simulink model "P2_SIL_Model_Diag"  (R2016a)
settings: Solver=ode2  StartTime=0.0  StopTime=Cycle_End  RelTol=1e-3
undefined symbols (not defined in the file): air, APP1_OOR, APP2_OOR, APP_Conversion_IN, APP_Mismatch, bms_inletair_temp, bms_maxchargecurrent, bms_maxdischargecurrent, BMS_Notfallkuehlung, BPP_Flt, cal, clt, ClutchEngag, CrankRequest, dcdc, eng, Engine, EngOverTemp, ENGTRQ_MSMCH_Degraded_CP, ENGTRQ_MSMCH_ErrCritical_CP, ENGTRQ_MSMCH_LimpHome_CP, EngTrqMismatch, env, ess, ESS, ESSOverTemp, fd, FFD, g, gb, Grade, IMG, KeyPos_Flt, KeyPosition, lib_APP_Conversion_IN, lib_ESS_plant_V1_2, lib_OBC_Manager, LossCAN, max_vehicle_rad_air_flow, MCUOverTemp, mot, MotDirMismatch, MotOverTemp, MotTrqMismatch, mph2kph, mph2ms, NeutralGear, obc, OBC_Manager, ParkGear, PRNDL_Flt, ReverseGear, RFD, rho, ShiftLeverPosition, sigbuilder_block, Speed, t_amb, time, tloop ... (+2)
libraries: simulink x104, EC2_libraries x12, Diagnostic x11, lib_CANerror_Detect x3, Utility x1
(part 11 of 11)

== stateflow chart P2_SIL_Model_Diag/Controller/HSC/Powertrain Manager/PowertrainSUSD/Motor Wake up // Shutdown ==
  state MCU_Restart [commented out]
    en:MCU_State = 10;
    MCU_Wake = 0;
    Fault_Counter++;
    during: timer++;
  state MCU_Startup
    state MCU_Wake
      en:MCU_State = 0;
      MCU_Wake = 1;
      MCUFault = 0;
      %Inverter_Enable = 0;
      Inverter_Discharge=0;
      MCU_ShtdwnRdy=0;
      Fault_Counter = 0;
    state MCU_Fault_1
      en:MCU_State = -1;
      MCUFault = 1;
    state MCU_Running
      en:MCU_State =3;
    state MCU_Enable
      en:MCU_State = 2;
      %Inverter_Enable = 1;
      during: timer++;
    state MCU_Ready
      en:MCU_State = 1;
    (default) -> MCU_Wake
    (junction 244) -> MCU_Fault_1 [order 2] : after(10,sec)
    (junction 244) -> MCU_Running [order 1] : [Inverter_Enabled]
    MCU_Enable -> (junction 244)
    MCU_Wake -> MCU_Ready : [CAN_Acc]
    MCU_Ready -> MCU_Enable : [RdyToDrv&&EnableInverter]
        | {timer = 0;}
  state MCU_Shutdown
    state MCU_Disable
      en:MCU_State = 8;
      during: timer++;
    state MCU_RdyForShtDwn
      en:MCU_State = 6;
      MCU_ShtdwnRdy=1;
    state MCU_Discharge_Bus
      en:MCU_State = 7;
      Inverter_Discharge=1;
    state MCU_Shtdwn_Cmplt
      en:MCU_State = 9;
      MCU_Wake = 0;
    state MCU_Fault_3
      en:MCU_State = -3;
      MCUFault = 1;
    (default) -> MCU_RdyForShtDwn : {timer = 0;}
    MCU_RdyForShtDwn -> MCU_Discharge_Bus : [HVDischarge]
    MCU_Discharge_Bus -> MCU_Disable : [!HVDischarge &&!EnableInverter]
        | {timer=0;}
    MCU_Disable -> (junction 247)
    (junction 247) -> MCU_Fault_3 [order 2] : after(10,sec)
    (junction 247) -> MCU_Shtdwn_Cmplt [order 1] : [!Inverter_Enabled]
  MCU_Restart -> MCU_Startup [commented out] : [timer > Restart_Time]
      | {timer = 0;}
  MCU_Startup -> MCU_Restart [commented out] : [(MCU_State==3 && !Inverter_Enabled || MCU_State==-1) && Fault_Counter<6]
      | {timer = 0;}
  MCU_Shutdown -> MCU_Startup : [RdyToDrv || RdyToChg]
  MCU_Startup -> MCU_Shutdown : [!RdyToDrv && !RdyToChg && Motor_Current < MaxShtdwnCrnt]
  (default) -> MCU_Shutdown
  data: MCU_State output int8; MCU_ShtdwnRdy output boolean; MCUFault output boolean; MCU_Wake output boolean; Inverter_Discharge output boolean; Inverter_Enable output boolean; RdyToDrv input boolean; RdyToChg input boolean; HVDischarge input boolean; Inverter_Response_Time input double; Restart_Time input double; MaxShtdwnCrnt input double; Inverter_Enabled input boolean; timer local double; Fault_Counter local double; Motor_Current input; CAN_Acc input boolean; EnableInverter input

== stateflow chart P2_SIL_Model_Diag/Controller/HSC/Powertrain Manager/Torque Distribution/Supervisory  Control  Logic1 ==
  state VehOffOrAcc
    en:
    powerMode = 0;
    EnablePrplsn = 0;
    HV_Req=0;
    closeMaincReq=0;
  state VehOn
    en:
    powerMode = 1;
    HV_Req=1;
    closeMaincReq = 1;
  state VehShutdown
    en:
    powerMode = 1;
    EnablePrplsn = 0;
    EngOnReq = 0;
    MotTrqReq = 0;
    EngAppReq = 0;
    EnableInverter=0;
  state EnablePropulsion
    en:
    EnablePrplsn = 1;
    EnableInverter = 1;
  state VehReady
    en:
    powerMode = 2;
    note: CD Limited
        | Engine Limited
    note: Fault detected?
    state Transition2
      en:
      MotTrqReq = 0;
      EngAppReq = 0;
      ClutchEngage = 1;
      state EngApp = SyncCtrl(EngSpeed,MotorSpeed) [function]
      state EngStart
        en: EngOnReq = 1;
      (default) -> VehReady.Transition2.EngStart : [VehicleSpeed < 1 && TransEstGear == 15]
    state CD_Limited
      en:
      EngOnReq = 0;
      mode=6;
      du:
      MotTrqReq = MotTrqCalc1(drvAPP,BrkPdlPos,VehicleSpeed,ShftLvrPos,MotSpd,DrvIntdAxleTrq,TransRatio,MotTrqMismchDegraded,MotTrqMismchLimp,essTempRange,MCUTempRange,MotorTempRange);
      EngAppReq = 0;
      state T = MotTrqCalc1(APP,BPP,VehSpd,ShftLvrPos,MotSpeed,DrvIntdAxleTrq,TransRatio,MotTrqMismchDegraded,MotTrqMismchLimp,essTempRange,MCUTempRange,MotorTempRange) [function]
    state CD_Mode
      en:
      EngOnReq = 0;
      mode=1;
      du:
      MotTrqReq = MotTrqCalc1(drvAPP,BrkPdlPos,VehicleSpeed,ShftLvrPos,MotSpd,DrvIntdAxleTrq,TransRatio,eSystemStatus);
      EngAppReq = 0;
      state T = MotTrqCalc(APP,BPP,VehSpd,Shifter,MotSpeed) [function] [commented out]
      state T = MotTrqCalc1(APP,BPP,VehSpd,ShftLvrPos,MotSpeed,DrvIntdAxleTrq,TransRatio,eSystemStatus) [function]
    state Sport_Mode
      en:
      mode=4;
      EngOnReq = 1;
      EngTrq = 0;
      du:
      MotTrqReq = MotTrqCalc(drvAPP,BrkPdlPos,VehicleSpeed,ShftLvrPos,MotSpd,DrvIntdAxleTrq,TransRatio);
      EngTrq = EngTrqCalc(drvAPP,EngSpd,ShftLvrPos,DrvIntdAxleTrq,TransRatio);
      EngAppReq = EngTrq2EngApp(EngTrq);
      state T = MotTrqCalc(APP,BPP,VehSpd,Shifter,MotSpeed,DrvIntdAxleTrq,TransRatio) [function]
      state T = EngTrqCalc(APP,EngSpeed,Shifter,DrvIntdAxleTrq,TransRatio) [function]
      state APP = EngTrq2EngApp(Trq) [function]
    state Transition
      en:
      MotTrqReq = 0;
      EngAppReq = 0;
      state EngStart1
        en: EngOnReq = 1;
      state EngApp = SyncCtrl(EngSpeed,MotorSpeed) [function]
      state EngageClutch
        en:
        ClutchEngage = 1;
      state EngSpdSync
        du:
        EngAppReq = SyncCtrl(EngSpd,MotSpd);
      state EngStart
        en: EngOnReq = 1;
      state EngageClutch1
        en:
        ClutchEngage = 1;
      (default) -> (junction 148)
      (junction 148) -> VehReady.Transition.EngStart1 [order 2] : [VehicleSpeed >= 1]
      (junction 148) -> VehReady.Transition.EngageClutch [order 1] : [VehicleSpeed < 1]
      VehReady.Transition.EngStart1 -> VehReady.Transition.EngSpdSync : [EngRunAtv]
      VehReady.Transition.EngageClutch -> VehReady.Transition.EngStart : [ClutchEngage == 1]
      VehReady.Transition.EngSpdSync -> VehReady.Transition.EngageClutch1 : [abs(EngSpd - MotSpd) < 20]
    state Engine_Limited [commented out]
    state Eng_Only_Mode
      en:
      EngOnReq = 1;
      mode=5;
      du:
      MotTrqReq = 0;
      EngTrq = EngTrqCalc(drvAPP,EngSpd,ShftLvrPos,DrvIntdAxleTrq,TransRatio,iceSystemStatus,EngTrqMismchDegraded,EngTrqMismchLimp,Eng_TempRange);
      EngAppReq = EngTrq2EngApp(EngTrq);
      closeMaincReq=0;
      state T = EngTrqCalc(APP,EngSpeed,Shifter,DrvIntdAxleTrq,TransRatio,iceSystemStatus,EngTrqMismchDegraded,EngTrqMismchLimp,Eng_TempRange) [function]
      state APP = EngTrq2EngApp(Trq) [function]
    state CS_Mode
      note: //*Removed transition : after(5,sec)[SoC > CS_SOC_MAX || VehicleSpeed < 50 && SoC > (CS_SOC_MIN+5)||VehicleSpeed > 5 && BrkPdlPos > 40]
      state Engine_Drive
        en:
        mode=2;
        du:
        EngTrq = EngTrqCalc(EngSpd,drvAPP,VehicleSpeed,ShftLvrPos,DrvIntdAxleTrq,TransRatio);
        EngAppReq = EngTrq2EngApp(EngTrq,TransRatio);
        MotTrqReq = MotTrqCalc2(drvAPP,BrkPdlPos,EngTrq,VehicleSpeed,ShftLvrPos,DrvIntdAxleTrq,TransRatio,Chg,SoC);
        Chg=ChgCalc(EngSpd,drvAPP,VehicleSpeed,DrvIntdAxleTrq,TransRatio);
        state APP = EngTrq2EngApp(Trq,TransRatio) [function]
        state Trq = EngTrqCalc(EngSpeed,APP,VehSpd,ShftLvrPos,DrvIntdAxleTrq,TransRatio) [function]
        state MotTrq = MotTrqCalc1(APP,BPP,EngTrq,VehSpd,ShftLvrPos,DrvIntdAxleTrq,TransRatio,Chg,SoC) [function] [commented out]
        state Chg = ChgCalc(EngSpeed,APP,VehSpd,DrvIntdAxleTrq,TransRatio) [function]
        state MotTrq = MotTrqCalc2(APP,BPP,EngTrq,VehSpd,ShftLvrPos,DrvIntdAxleTrq,TransRatio,Chg,SoC) [function]
        state MotTrq = MotTrqCalc(APP,BPP,EngTrq,VehSpd,ShftLvrPos,DrvIntdAxleTrq,TransRatio) [function] [commented out]
      state Motor_Drive
        en:
        ClutchEngage = 0;
        EngOnReq = 0;
        mode=3;
        du:
        MotTrqReq = MotTrqCalc1(drvAPP,BrkPdlPos,VehicleSpeed,ShftLvrPos,MotSpd,DrvIntdAxleTrq,TransRatio);
        EngAppReq = 0;
        state T = MotTrqCalc1(APP,BPP,MotSpeed,VehSpd,DrvIntdAxleTrq,TransRatio,ShftLvrPos) [function]
      state Transition
        en:
        EngAppReq = 0;
        du:
        MotTrqReq = MotTrqCalc(drvAPP,BrkPdlPos,VehicleSpeed,ShftLvrPos,MotSpd,DrvIntdAxleTrq,TransRatio);
        EngAppReq = 0;
        state MotTrq = MotTrqCalc(APP,BPP,EngTrq,VehSpd,DrvIntdAxleTrq,TransRatio,ShftLvrPos) [function]
        state EngApp = SyncCtrl(EngSpeed,MotorSpeed) [function]
        state EngStart
          en: EngOnReq = 1;
        state EngSpdSync
          du:
          EngAppReq = SyncCtrl(EngSpd,MotSpd);
        state EngageClutch
          en:
          ClutchEngage = 1;
        (default) -> VehReady.CS_Mode.Transition.EngStart
        VehReady.CS_Mode.Transition.EngStart -> VehReady.CS_Mode.Transition.EngSpdSync : [EngRunAtv]
        VehReady.CS_Mode.Transition.EngSpdSync -> VehReady.CS_Mode.Transition.EngageClutch : [abs(EngSpd - MotSpd) < 20]
      (default) -> Engine_Drive
      VehReady.CS_Mode.Transition -> Engine_Drive [commented out] : [ClutchEngage == 1]
      Motor_Drive -> VehReady.CS_Mode.Transition [commented out] : after(5,sec)[SoC < CS_SOC_MIN && BrkPdlPos == 0]
    state Transition1
      en:
      MotTrqReq = 0;
      EngAppReq = 0;
      state EngStart1
        en: EngOnReq = 1;
      state EngApp = SyncCtrl(EngSpeed,MotorSpeed) [function]
      state EngageClutch
        en:
        ClutchEngage = 1;
      state EngSpdSync
        du:
        EngAppReq = SyncCtrl(EngSpd,MotSpd);
      state EngageClutch1
        en:
        ClutchEngage = 1;
      (default) -> (junction 157)
      (junction 157) -> VehReady.Transition1.EngStart1 [order 2] : [ClutchEngage == 0]
      (junction 157) -> VehReady.Transition1.EngageClutch [order 1] : [ClutchEngage == 1]
      VehReady.Transition1.EngStart1 -> VehReady.Transition1.EngSpdSync : [EngRunAtv]
      VehReady.Transition1.EngSpdSync -> VehReady.Transition1.EngageClutch1 : [abs(EngSpd - MotSpd) < 20]
    (default) -> CD_Mode
    CD_Mode -> CD_Limited [order 3] : [eSystemStatus==1]
    CD_Mode -> Transition2 [order 2] : [SportModeEnabled == 1&&iceSystemStatus == 2 && ...
        | eSystemStatus == 2]
    Transition2 -> Sport_Mode : [EngRunAtv]
    CD_Limited -> CD_Mode : [eSystemStatus==2]
    Sport_Mode -> CD_Mode [commented out]
    Eng_Only_Mode -> CD_Mode [order 1] : [(SoC > CD_SOC_MIN && ...
        | eSystemStatus == 2) || ...
        | (iceSystemStatus == 0&&eSystemStatus)]
    CD_Mode -> Eng_Only_Mode [order 4] : [(SoC < CD_SOC_MIN && ...
        | iceSystemStatus == 2)||(iceSystemStatus&&eSystemStatus == 0)]
    CS_Mode -> CD_Mode [order 1] : [(SoC > CD_SOC_MIN||...
        | LossECMCAN == 1 ||...
        | APPFault == 1&&eSystemStatus == 2) || ...
        | iceSystemStatus == 0]
    CD_Mode -> VehReady.Transition [order 1] : [SoC <CS_SOC_MIN&&iceSystemStatus == 2 && ...
        | eSystemStatus == 2]
    Eng_Only_Mode -> Sport_Mode [commented out]
    Sport_Mode -> Eng_Only_Mode [commented out]
    VehReady.Transition -> CS_Mode : after(1,sec)
        | [ClutchEngage==1&&EngRunAtv == 1]
    CS_Mode -> Eng_Only_Mode [order 2] : [(SoC<.02&&iceSystemStatus==2)||(eSystemStatus==0&&iceSystemStatus)]
    Eng_Only_Mode -> CS_Mode [order 2] : [SoC <CS_SOC_MIN&&SoC>.02&&eSystemStatus&&iceSystemStatus]
  (default) -> VehOffOrAcc
  VehOffOrAcc -> VehOn : [KeyPos >= 1&&(eSystemStatus||iceSystemStatus)]
  VehOn -> VehOffOrAcc [order 2] : [KeyPos < 1&&(eSystemStatus==0&&iceSystemStatus==0)]
  VehOn -> EnablePropulsion [order 1] : [KeyPos>=3&&BrkPdlPos>20&&ShftLvrPos==1]
  VehShutdown -> VehOffOrAcc : after(1,sec)[!InverterEnabled]
  EnablePropulsion -> VehReady : [InverterEnabled == 1]
  VehReady -> VehShutdown : [KeyPos < 2&&ShftLvrPos==1||(eSystemStatus==0&&iceSystemStatus==0)]
  data: EngSpeed function_input; EngApp function_output; MotorSpeed function_input; T function_output; APP function_input; BPP function_input; VehSpd function_input; ShftLvrPos function_input; MotSpeed function_input; DrvIntdAxleTrq function_input; TransRatio function_input; MotTrqMismchDegraded function_input; MotTrqMismchLimp function_input; essTempRange function_input; MCUTempRange function_input; MotorTempRange function_input; T function_output double size=1; APP function_input double size=1; BPP function_input double size=1; VehSpd function_input double size=1; Shifter function_input double size=1; MotSpeed function_input double size=1; T function_output; APP function_input; BPP function_input; VehSpd function_input; ShftLvrPos function_input; MotSpeed function_input; DrvIntdAxleTrq function_input; TransRatio function_input; eSystemStatus function_input; T function_output; APP function_input; BPP function_input; VehSpd function_input; Shifter function_input; MotSpeed function_input; DrvIntdAxleTrq function_input; TransRatio function_input; APP function_input; EngSpeed function_input; T function_output; Shifter function_input; DrvIntdAxleTrq function_input; TransRatio function_input; Trq function_input; APP function_output; temp local double; EngSpeed function_input; EngApp function_output; MotorSpeed function_input; APP function_input; EngSpeed function_input; T function_output; Shifter function_input; DrvIntdAxleTrq function_input; TransRatio function_input; iceSystemStatus function_input; EngTrqMismchDegraded function_input; EngTrqMismchLimp function_input; Eng_TempRange function_input; Trq function_input; APP function_output; Trq function_input; APP function_output; TransRatio function_input; Trq function_output; EngSpeed function_input; APP function_input; VehSpd function_input; ShftLvrPos function_input; DrvIntdAxleTrq function_input; TransRatio function_input; APP function_input double size=1; MotTrq function_output double size=1; BPP function_input double size=1; EngTrq function_input double size=1; VehSpd function_input double size=1; ShftLvrPos function_input double size=1; DrvIntdAxleTrq function_input double size=1; TransRatio function_input double size=1; Chg function_input double size=1; SoC function_input double size=1; EngSpeed function_input; APP function_input; VehSpd function_input; DrvIntdAxleTrq function_input; TransRatio function_input; Chg function_output; APP function_input; MotTrq function_output; BPP function_input; EngTrq function_input; VehSpd function_input; ShftLvrPos function_input; DrvIntdAxleTrq function_input; TransRatio function_input; Chg function_input; SoC function_input; APP function_input double size=1; MotTrq function_output double size=1; BPP function_input double size=1; EngTrq function_input double size=1; VehSpd function_input double size=1; ShftLvrPos function_input double size=1; DrvIntdAxleTrq function_input double size=1; TransRatio function_input double size=1; APP function_input; BPP function_input; MotSpeed function_input; VehSpd function_input; DrvIntdAxleTrq function_input; TransRatio function_input; T function_output; ShftLvrPos function_input; APP function_input; MotTrq function_output; BPP function_input; EngTrq function_input; VehSpd function_input; DrvIntdAxleTrq function_input; TransRatio function_input; ShftLvrPos function_input; EngSpeed function_input; EngApp function_output; MotorSpeed function_input; data local double; EngSpeed function_input; EngApp function_output; MotorSpeed function_input; TransEstGear input int8; SportModeEnabled input boolean; mode output int8; powerMode output int8; closeMaincReq output double; EnablePrplsn output boolean; KeyPos input int8; BrkPdlPos input double; drvAPP input double; VehicleSpeed input double; EngSpd input double; MotSpd input double; ShftLvrPos input int8; ClutchEngage output boolean; EngAppReq output double; EngOnReq output boolean; MotTrqReq output double; EnableInverter output boolean; InverterEnabled input boolean; CD_SOC_MIN input double; CS_SOC_MIN input double; CS_SOC_MAX input double; EngRunAtv input boolean; SoC input double; ESSOverheat input double; LossECMCAN input boolean; APPFault input boolean; EngTrq output double; DrvIntdAxleTrq input double; TransRatio input double; HV_Req output double; Chg output double; eSystemStatus input double; iceSystemStatus input double; MotTrqMismchDegraded input boolean; MotTrqMismchLimp input boolean; EngTrqMismchDegraded input boolean; EngTrqMismchLimp input boolean; essTempRange input double; MCUTempRange input double; MotorTempRange input double; Eng_TempRange input double

== stateflow chart P2_SIL_Model_Diag/Controller/HSC/Driver_Requests/Vehicle_Shutdown/HCU_Shutdown ==
  state HCU_On
    entry:
    HCUStatus = 0;
    HCU_ON = 1;
  state Power_Down
    state PowerDownComponentsWait
      entry: HCUStatus = 1;
      timer = 1;
      during: timer++;
    state Diagnostics_Record
      entry: HCUStatus = 2;
      timer = 1;
      during: timer++;
    state HCU_OFF
      entry: HCUStatus = 3;
      HCU_ON = 0;
    (default) -> PowerDownComponentsWait
    PowerDownComponentsWait -> Diagnostics_Record : [DisableComponents]
    Diagnostics_Record -> HCU_OFF : [timer>= DiagUSBTimerMax]
  (default) -> HCU_On
  Power_Down -> HCU_On : [Key_Position >= 1 || Plugged]
  HCU_On -> Power_Down : [Key_Position==0 && !Plugged]
  data: DisableComponents input; DiagUSBTimerMax input; Key_Position input; Plugged input; HCUStatus output double; HCU_ON output boolean; timer local double

== stateflow chart P2_SIL_Model_Diag/Controller/HSC/Powertrain Manager/PowertrainSUSD/Crank Engine/Crank_Stop_Engine ==
  state Eng_Off
    entry:
    EngState = 0;
    CrankCmd = 0;
  state Engine_On
    state Crank_Engine
      entry:
      EngState = 1;
      CrankCmd = 1;
      during: timer++;
    state Engine_Running
      entry:
      EngState = 2;
      CrankCmd = 0;
      timer=0;
    (default) -> Crank_Engine
    Crank_Engine -> Engine_Running : [EngRunAtv]
  (default) -> Eng_Off
  Engine_On -> Eng_Off : [((EngState==1 && timer > CrankEngTime) || (SysPwrMd < 2) || (EngState==2 && !EngRunAtv)) && ClutchEngage==0]
  Eng_Off -> Engine_On : [EnablePrplsn && SysPwrMd == 3 && ClutchEngage==0]
      | {timer = 0;}
  data: SysPwrMd input; ClutchEngage input; CrankCmd output; EnablePrplsn input boolean; EngRunAtv input boolean; EngState output double; CrankEngTime input; timer local double

== stateflow chart P2_SIL_Model_Diag/Controller/HSC/Camaro Fault Detection/Component Diagnostic/ESS Component Diagnostic/BMS_CompDiag ==
  state BMSOnline
    en:BMS_Status=2
  state BMSLimited
    en: BMS_Status=1
  state BMSOffline
    en: BMS_Status=0
  BMSOnline -> BMSLimited
  BMSLimited -> BMSOnline [order 1] : [BMS_essTemp_[degC]_SigValid]
  BMSLimited -> BMSOffline [order 2]
  BMSOffline -> BMSLimited : [essTempRange==4 &&BMS_RollingAliveActive_SigValid &&BMS_contactorsFailed_SigValid]
  (default) -> BMSOffline
  data: BMS_RollingAliveActive_SigValid input; BMS_contactorsFailed_SigValid input; BMS_essTemp__degC__SigValid input; BMS_Status output

== stateflow chart P2_SIL_Model_Diag/Controller/HSC/Camaro Fault Detection/Component Diagnostic/ESS Component Diagnostic/BMS_CompDiag1 ==
  state BMS_Offline
    en: BMS_Status=0;
  state BMS_Online
    en:BMS_Status=2;
  state BMS_Limited
    en: BMS_Status=1;
  BMS_Online -> BMS_Offline [order 2] : [~BMS_RollingAliveActive_SigValid||~BMS_contactorsFailed_SigValid||~BMS_essSOC_0_1_SigValid|| ~ess_GroundFault]
  BMS_Offline -> BMS_Online [order 1] : [BMS_RollingAliveActive_SigValid&&BMS_contactorsFailed_SigValid&&BMS_essTemp_SigValid&&ClearFault&&BMS_essSOC_0_1_SigValid&&ess_GroundFault&&essCur_A_SigValid]
  (default) -> BMS_Offline
  BMS_Limited -> BMS_Offline [order 2] : [~BMS_RollingAliveActive_SigValid||~BMS_contactorsFailed_SigValid]
  BMS_Offline -> BMS_Limited [order 2] : [BMS_RollingAliveActive_SigValid &&...
      | BMS_contactorsFailed_SigValid && ~BMS_essTemp_SigValid|| ~BMS_essSOC_0_1_SigValid]
  BMS_Online -> BMS_Limited [order 1] : [~BMS_essTemp_SigValid|| ~BMS_essSOC_0_1_SigValid]
  BMS_Limited -> BMS_Online [order 1] : [BMS_essTemp_SigValid||ClearFault||BMS_essSOC_0_1_SigValid]
  data: BMS_RollingAliveActive_SigValid input; BMS_contactorsFailed_SigValid input; BMS_essTemp_SigValid input; BMS_Status output; BMS_essSOC_0_1_SigValid input; essCur_A_SigValid input; ess_GroundFault input; ClearFault input

== stateflow chart P2_SIL_Model_Diag/Controller/HSC/Camaro Fault Detection/Component Diagnostic/Motor Component Diagnostic/MCU_CompDiag ==
  state MCU_Offline
    en: MCU_Status=0;
  state MCU_Online
    en:MCU_Status=2;
  state MCU_Limited
    en: MCU_Status=1;
  MCU_Online -> MCU_Offline [order 2] : [~MCU_RollingAliveActive||~Motor_TrqCmd_Nm_SigValid||...
      | ~Motor_Speed_rpm_SigValid||~Torq_Feedback_SigValid||(MCU_torq_mismch==1)...
      | ||~Dir_Command_SigValid||~Dir_feedback_SigValid||Dir_Mismch==1||~dc_bus_voltage_SigValid...
      | ||Voltage_Mismch==1||~MotorTemp_degC_SigValid||...
      | ~MCUTemp_degC_SigValid]
  MCU_Offline -> MCU_Online [order 1] : [MCU_RollingAliveActive&&MCUTemp_degC_SigValid &&...
      | MotorTemp_degC_SigValid&&Motor_TrqCmd_Nm_SigValid...
      | &&Motor_Speed_rpm_SigValid&&Torq_Feedback_SigValid&&(MCU_torq_mismch==0)...
      | &&Dir_Command_SigValid&&Dir_feedback_SigValid&&Dir_Mismch==0&&dc_bus_voltage_SigValid...
      | &&Voltage_Mismch==0]
  (default) -> MCU_Offline
  MCU_Limited -> MCU_Offline [order 2] : [~MCU_RollingAliveActive||~Motor_TrqCmd_Nm_SigValid...
      | ||~Motor_Speed_rpm_SigValid||~Torq_Feedback_SigValid||(MCU_torq_mismch==1)...
      | ||~Dir_Command_SigValid||~Dir_feedback_SigValid||Dir_Mismch==1||~dc_bus_voltage_SigValid...
      | ||Voltage_Mismch==1|| ~MotorTemp_degC_SigValid||...
      | ~MCUTemp_degC_SigValid]
  MCU_Offline -> MCU_Limited [order 2] : [MCU_RollingAliveActive...
      | &&Motor_TrqCmd_Nm_SigValid &&Motor_Speed_rpm_SigValid...
      | &&Torq_Feedback_SigValid&&(MCU_torq_mismch==0)...
      | &&Dir_Command_SigValid&&Dir_feedback_SigValid&&Dir_Mismch==0&&dc_bus_voltage_SigValid...
      | &&Voltage_Mismch==0&&MotorTemp_degC_SigValid &&MCUTemp_degC_SigValid&&(MCUTempRange==1||MCUTempRange==3)||...
      | (MotTempRange==1||MotTempRange==3)]
  MCU_Online -> MCU_Limited [order 1] : [(MCUTempRange==1||MCUTempRange==3)||...
      | (MotTempRange==1||MotTempRange==3)]
  MCU_Limited -> MCU_Online [order 1] : [MotorTemp_degC_SigValid&&MCUTemp_degC_SigValid&&...
      | (MCUTempRange==2)&&...
      | (MotTempRange==2)]
  data: MCU_RollingAliveActive input; MCUTemp_degC_SigValid input; MotorTemp_degC_SigValid input; Motor_TrqCmd_Nm_SigValid input; Torq_Feedback_SigValid input; MCU_torq_mismch input; Motor_Speed_rpm_SigValid input; MCUTempRange input; MotTempRange input; MCU_Status output; Dir_Command_SigValid input; Dir_feedback_SigValid input; Dir_Mismch input; dc_bus_voltage_SigValid input; Voltage_Mismch input

== stateflow chart P2_SIL_Model_Diag/Controller/HSC/Camaro Fault Detection/Signal Diagnostic/Driver Signal Diagnostic/AccPedalValidity ==
  state SignalHigh
    en: signalValid=0;
  state SignalInRange
  state SignalLow
    en:signalValid=0;
  SignalHigh -> SignalInRange : [signalValue<=100]
  SignalInRange -> SignalHigh [order 1] : [signalValue>102]
  SignalInRange -> SignalInRange [order 3] : [clearFaults==1]
      | {signalValid=1;}
  (default) -> SignalInRange : {signalValid=1;}
  SignalLow -> SignalInRange : [signalValue>0]
  SignalInRange -> SignalLow [order 2] : [signalValue<-2]
  data: clearFaults input; signalValue input; signalValid output

== stateflow chart P2_SIL_Model_Diag/Controller/HSC/Camaro Fault Detection/Component Diagnostic/Engine Component Diagnostic/ECM_CompDiag ==
  state ECM_Offline
    en: ECM_Status=0;
  state ECM_Online
    en:ECM_Status=2;
  state ECM_Limited
    en: ECM_Status=1;
  ECM_Online -> ECM_Offline [order 2] : [~ECM_RollingAliveActive||~engTrqCmdRecvd_SigValid||...
      | ~Engine_Speed_rpm_SigValid||Eng_TempRange_123==3||Eng_Torq_Msmch==1||ClearFault==0]
  (default) -> ECM_Offline
  ECM_Offline -> ECM_Online [order 1] : [ECM_RollingAliveActive&&engTrqCmdRecvd_SigValid &&...
      | Engine_Speed_rpm_SigValid&&ClearFault&&Eng_TempRange_123==1&&Eng_Torq_Msmch==0&&ClearFault]
  ECM_Limited -> ECM_Offline [order 2] : [~ECM_RollingAliveActive||~engTrqCmdRecvd_SigValid||~Engine_Speed_rpm_SigValid|| Eng_TempRange_123==3||Eng_Torq_Msmch==1]
  ECM_Offline -> ECM_Limited [order 2] : [ECM_RollingAliveActive...
      | &&engTrqCmdRecvd_SigValid &&Engine_Speed_rpm_SigValid...
      | &&Eng_Torq_Msmch==0&&[Eng_TempRange_123==2 ]]
  ECM_Limited -> ECM_Online [order 1] : [Eng_TempRange_123==1&&Eng_Torq_Msmch==0]
  ECM_Online -> ECM_Limited [order 1] : [ECM_RollingAliveActive...
      | &&engTrqCmdRecvd_SigValid &&Engine_Speed_rpm_SigValid...
      | &&Eng_Torq_Msmch==0&&(Eng_TempRange_123==2 )]
  data: ECM_RollingAliveActive input; engTrqCmdRecvd_SigValid input; Eng_Torq_Msmch input; Engine_Speed_rpm_SigValid input; Eng_TempRange_123 input; ECM_Status output; ClearFault input

== stateflow chart P2_SIL_Model_Diag/Controller/HSC/Camaro Fault Detection/Signal Diagnostic/Driver Signal Diagnostic/AccPedalValidity1 ==
  state SignalHigh
    en: signalValid=0;
  state SignalInRange
  state SignalLow
    en:signalValid=0;
  SignalHigh -> SignalInRange : [signalValue<=100]
  SignalInRange -> SignalHigh [order 1] : [signalValue>102]
  SignalInRange -> SignalInRange [order 3] : [clearFaults==1]
      | {signalValid=1;}
  (default) -> SignalInRange : {signalValid=1;}
  SignalLow -> SignalInRange : [signalValue>0]
  SignalInRange -> SignalLow [order 2] : [signalValue<-2]
  data: clearFaults input; signalValue input; signalValid output

== stateflow chart P2_SIL_Model_Diag/Controller/HSC/Camaro Fault Detection/Component Diagnostic/Driver Input Diagnostic/Driver_Input_Diag ==
  state Driver_Input_Offline
    en: Driver_Input_Status=0;
  state Driver_Input_Online
    en: Driver_Input_Status=1;
  (default) -> Driver_Input_Offline
  Driver_Input_Online -> Driver_Input_Offline : [~APP_Valid|| ~Drv_BPP_SigValid||~KeyPos||~PRNDL]
  Driver_Input_Offline -> Driver_Input_Online : [APP_Valid&&Drv_BPP_SigValid&&KeyPos&&PRNDL]
  data: APP_Valid input; Drv_BPP_SigValid input; KeyPos input; Driver_Input_Status output; PRNDL input

== stateflow chart P2_SIL_Model_Diag/Controller/HSC/Camaro Fault Detection/Signal Diagnostic/ESS Signal Diagnostic/Rolling Alive Counter Detection/Chart ==
  state Off
    en:flag=0;
  state Alive
    en:flag=1;
  state Dead
    en:flag=0;
  Alive -> Alive [order 1] : after(CycleTime-tloop,sec)
      | [PulseDetect==1]
  (default) -> Off
  Off -> Alive : [PulseDetect==1]
  Alive -> Dead [order 2] : after(CycleTime,sec)
  data: PulseDetect input; CycleTime input; flag output; tloop input

== stateflow chart P2_SIL_Model_Diag/Controller/HSC/Camaro Fault Detection/Signal Diagnostic/ESS Signal Diagnostic/essSOC_0_1Range ==
  state aboveMax
    en: essSOCRange=3;
  state NormalRange
    en: essSOCRange=2;
  state LowRange
    en:essSOCRange=1;
  state BelowNormal
    en: essSOCRange=0;
  aboveMax -> NormalRange : [signalValue<0.95]
  NormalRange -> aboveMax [order 1] : [signalValue>=0.95]
  NormalRange -> NormalRange [order 3] : [clearFaults==1]
      | {essSOCRange=2;}
  (default) -> NormalRange
  LowRange -> NormalRange [order 1] : [signalValue>0.3]
  NormalRange -> LowRange [order 2] : [signalValue<=0.3&&signalValue>0.15]
  LowRange -> BelowNormal [order 2] : [signalValue<=0.15]
  BelowNormal -> LowRange : [signalValue>0.15]
  data: clearFaults input; signalValue input; data local; essSOCRange output

== stateflow chart P2_SIL_Model_Diag/Controller/HSC/Camaro Fault Detection/Component Diagnostic/Transmission Component Diagnostic/TCM_CompDia ==
  state TCM_Limited
    en: TCM_Status=1;
  state TCM_Offline
    en: TCM_Status=0;
  state TCM_Online
    en: TCM_Status=2;
  (default) -> TCM_Offline
  TCM_Offline -> TCM_Limited [commented out]
  TCM_Limited -> TCM_Offline [commented out]
  TCM_Online -> TCM_Offline : [~TCMRollingAliveActive_SigValid||~LvrPosTrnsShft_SigValid||~TransEstGear_SigValid||~LockupCmd_SigValid]
  TCM_Offline -> TCM_Online : [TCMRollingAliveActive_SigValid&&LvrPosTrnsShft_SigValid&&TransEstGear_SigValid&&LockupCmd_SigValid]
  TCM_Limited -> TCM_Online [commented out]
  TCM_Online -> TCM_Limited [commented out]
  data: TCM_Status output; TCMRollingAliveActive_SigValid input; LvrPosTrnsShft_SigValid input; TransEstGear_SigValid input; LockupCmd_SigValid input

== stateflow chart P2_SIL_Model_Diag/Controller/HSC/Camaro Fault Detection/Signal Diagnostic/ESS Signal Diagnostic/essTsignalRange ==
  state AboveMax
    en: essTempRange=4;
  state HighRange
    en: essTempRange=3;
  state NormalRange
    en: essTempRange=2;
  state LowRange
    en:essTempRange=1;
  state BelowNormal
    en: essTempRange=0;
  HighRange -> AboveMax [order 2] : [signalValue>55]
  AboveMax -> HighRange : [signalValue<55]
  HighRange -> NormalRange [order 1] : [signalValue<=30]
  NormalRange -> HighRange [order 1] : [signalValue>32]
  NormalRange -> NormalRange [order 3] : [clearFaults==1]
      | {essTempRange=2;}
  (default) -> NormalRange
  LowRange -> NormalRange [order 1] : [signalValue>=30]
  NormalRange -> LowRange [order 2] : [signalValue<0 ]
  LowRange -> BelowNormal [order 2] : [signalValue<-28]
  BelowNormal -> LowRange : [signalValue>28]
  data: clearFaults input; signalValue input; essTempRange output; data local

== stateflow chart P2_SIL_Model_Diag/Controller/HSC/Camaro Fault Detection/Signal Diagnostic/Engine Signal Diagnostic/Engine_Temp[DegC] ==
  state AboveMax
    en: EngTempRange=3;
  state HighRange
    en: EngTempRange=2;
  state NormalRange
    en: EngTempRange=1;
  HighRange -> AboveMax [order 2] : [Engine_Temp_DegC>120]
  AboveMax -> HighRange : [Engine_Temp_DegC<120]
  NormalRange -> HighRange [order 1] : [Engine_Temp_DegC>100&&Engine_Temp_DegC<120]
  HighRange -> NormalRange [order 1] : [Engine_Temp_DegC<=100]
  NormalRange -> NormalRange [order 2] : [clearFaults==1]
      | {EngTempRange=1;}
  (default) -> NormalRange
  data: clearFaults input; Engine_Temp_DegC input; EngTempRange output; data local

== stateflow chart P2_SIL_Model_Diag/Controller/HSC/Camaro Fault Detection/Component Diagnostic/Clutch Component Diagnostic/Clutch_CompDia ==
  state Clutch_Offline
    en: Clutch_Status=0;
  state Clutch_Online
    en: Clutch_Status=1;
  (default) -> Clutch_Offline
  Clutch_Offline -> Clutch_Online : [ClutchRollingAliveActive_SigValid&&Engage_Clutch_SigValid&&clt_plant_spd_out_SigValid&&~EngageFailed]
  Clutch_Online -> Clutch_Offline : [~ClutchRollingAliveActive_SigValid||~Engage_Clutch_SigValid||~clt_plant_spd_out_SigValid||EngageFailed]
  data: Clutch_Status output; ClutchRollingAliveActive_SigValid input; Engage_Clutch_SigValid input; clt_plant_spd_out_SigValid input; EngageFailed input

== stateflow chart P2_SIL_Model_Diag/Controller/HSC/Camaro Fault Detection/Component Diagnostic/Engine Component Diagnostic/Eng_Torq_MsmchLevel ==
  state Normal_Torque
    en: Eng_Torq_MsmchLevel==1
  state Creep_Torq_Allowed
    en: Eng_Torq_MsmchLvel==3
  state AboveMax
    en: Eng_Torq_MsmchLevel==4
  state Max_power_limited
    en: Eng_Torq_MsmchLvel==2
  (default) -> Normal_Torque
  AboveMax -> Normal_Torque [order 2] : [SignalValue<ENGTRQ_MSMCH_Degraded_CP]
  Creep_Torq_Allowed -> AboveMax [order 2] : [SignalValue>ENGTRQ_MSMCH_ErrCritical_CP]
  Max_power_limited -> Normal_Torque [order 1] : [SignalValue<ENGTRQ_MSMCH_Degraded_CP]
  Normal_Torque -> Max_power_limited [order 1] : [SignalValue>ENGTRQ_MSMCH_Degraded_CP&&...
      | SignalValue<ENGTRQ_MSMCH_LimpHome_CP]
  Normal_Torque -> AboveMax [order 2] : [SignalValue>ENGTRQ_MSMCH_ErrCritical_CP]
  AboveMax -> Creep_Torq_Allowed [order 1] : [SignalValue>ENGTRQ_MSMCH_LimpHome_CP&&SignalValue<ENGTRQ_MSMCH_ErrCritical_CP]
  Max_power_limited -> Creep_Torq_Allowed [order 2] : [SignalValue>ENGTRQ_MSMCH_LimpHome_CP&&SignalValue<ENGTRQ_MSMCH_ErrCritical_CP]
  Creep_Torq_Allowed -> Max_power_limited [order 1] : [SignalValue<ENGTRQ_MSMCH_LimpHome_CP&&SignalValue>ENGTRQ_MSMCH_Degraded_CP]
  data: SignalValue input; ENGTRQ_MSMCH_Degraded_CP parameter; ENGTRQ_MSMCH_LimpHome_CP parameter; Eng_Torq_MsmchLevel output; ENGTRQ_MSMCH_ErrCritical_CP parameter

== stateflow chart P2_SIL_Model_Diag/Controller/HSC/Camaro Fault Detection/Signal Diagnostic/Clutch Signal Diagnostic/Rolling Alive Counter Detection/Chart ==
  state Off
    en:flag=0;
  state Alive
    en:flag=1;
  state Dead
    en:flag=0;
  Alive -> Alive [order 1] : after(CycleTime-tloop,sec)
      | [PulseDetect==1]
  (default) -> Off
  Off -> Alive : [PulseDetect==1]
  Alive -> Dead [order 2] : after(CycleTime,sec)
  data: PulseDetect input; CycleTime input; flag output; tloop parameter

== stateflow chart P2_SIL_Model_Diag/Controller/HSC/Camaro Fault Detection/Signal Diagnostic/Motor Signal Diagnostic/Rolling Alive Counter Detection/Chart ==
  state Off
    en:flag=0;
  state Alive
    en:flag=1;
  state Dead
    en:flag=0;
  Alive -> Alive [order 1] : after(CycleTime-tloop,sec)
      | [PulseDetect==1]
  (default) -> Off
  Off -> Alive : [PulseDetect==1]
  Alive -> Dead [order 2] : after(CycleTime,sec)
  data: PulseDetect input; CycleTime input; flag output; tloop parameter

== stateflow chart P2_SIL_Model_Diag/Controller/HSC/Camaro Fault Detection/Signal Diagnostic/Motor Signal Diagnostic/Subsystem/MCUTsignalRange ==
  note: Temperature Range check :
      | 0 = below normal operation (<-40)
      | 1 = low range (-39 to 0)
      | 2 = normal range (0 to 80 C)
      | 3= high range (80 to 99)
      | 4= above max value allowed (>100)
  state AboveMax
    en: MCUTempRange=4;
  state HighRange
    en: MCUTempRange=3;
  state NormalRange
    en: MCUTempRange=2;
  state LowRange
    en:MCUTempRange=1;
  state BelowNormal
    en: MCUTempRange=0;
  HighRange -> AboveMax [order 2] : [signalValue>100]
  AboveMax -> HighRange : [signalValue<100]
  HighRange -> NormalRange [order 1] : [signalValue<80]
  NormalRange -> HighRange [order 1] : [signalValue>80]
  NormalRange -> NormalRange [order 3] : [clearFaults==1]
      | {MCUTempRange=2;}
  (default) -> NormalRange
  LowRange -> NormalRange [order 1] : [signalValue>0]
  NormalRange -> LowRange [order 2] : [signalValue<0 ]
  LowRange -> BelowNormal [order 2] : [signalValue<-40]
  BelowNormal -> LowRange : [signalValue>-40]
  data: clearFaults input; signalValue input; MCUTempRange output; data local

== stateflow chart P2_SIL_Model_Diag/Controller/HSC/Camaro Fault Detection/Signal Diagnostic/Motor Signal Diagnostic/Subsystem1/MotorTsignalRange ==
  note: Temperature Range check :
      | 0 = below normal operation (<-20)
      | 1 = low range (-19 to 0)
      | 2 = normal range (0 to 70 C)
      | 3= high range (71 to 149)
      | 4= above max value allowed (>150)
  state AboveMax
    en: MotorTempRange=4;
  state HighRange
    en: MotorTempRange=3;
  state NormalRange
    en: MotorTempRange=2;
  state LowRange
    en:MotorTempRange=1;
  state BelowNormal
    en: MotorTempRange=0;
  HighRange -> AboveMax [order 2] : [signalValue>150]
  AboveMax -> HighRange : [signalValue<150]
  HighRange -> NormalRange [order 1] : [signalValue<70]
  NormalRange -> HighRange [order 1] : [signalValue>70]
  NormalRange -> NormalRange [order 3] : [clearFaults==1]
      | {MotorTempRange=2;}
  (default) -> NormalRange
  LowRange -> NormalRange [order 1] : [signalValue>0]
  NormalRange -> LowRange [order 2] : [signalValue<0 ]
  LowRange -> BelowNormal [order 2] : [signalValue<-20]
  BelowNormal -> LowRange : [signalValue>-20]
  data: clearFaults input; signalValue input; MotorTempRange output; data local

== stateflow chart P2_SIL_Model_Diag/Controller/HSC/Camaro Fault Detection/Signal Generator /BMS_Signals/BMS_rollingAliveCnt/Rolling Alive Counter ==
  state RollingAliveCounter
    state Count1
      en: RollingAliveCnt=0
    state Count2
      en: RollingAliveCnt=1
    state Count3
      en: RollingAliveCnt=2
    state Count4
      en: RollingAliveCnt=3
    (default) -> Count1
    Count4 -> Count1 : after(0.01,sec)
    Count1 -> Count2 : after(0.01,sec)
    Count2 -> Count3 : after(0.01,sec)
    Count3 -> Count4 : after(0.01,sec)
  data: RollingAliveCnt output double

== stateflow chart P2_SIL_Model_Diag/Controller/HSC/Camaro Fault Detection/Signal Generator /Clutch_Signals/Clutch_Rolling/Rolling Alive Counter1 ==
  state RollingAliveCounter
    state Count1
      en: RollingAliveCnt=0
    state Count2
      en: RollingAliveCnt=1
    state Count3
      en: RollingAliveCnt=2
    state Count4
      en: RollingAliveCnt=3
    (default) -> Count1
    Count4 -> Count1 : after(0.01,sec)
    Count1 -> Count2 : after(0.01,sec)
    Count2 -> Count3 : after(0.01,sec)
    Count3 -> Count4 : after(0.01,sec)
  data: RollingAliveCnt output double

== stateflow chart P2_SIL_Model_Diag/Controller/HSC/Camaro Fault Detection/Signal Generator /ECM_Signals/ECM_CAN_Rolling/Rolling Alive Counter1 ==
  state RollingAliveCounter
    state Count1
      en: RollingAliveCnt=0
    state Count2
      en: RollingAliveCnt=1
    state Count3
      en: RollingAliveCnt=2
    state Count4
      en: RollingAliveCnt=3
    (default) -> Count1
    Count4 -> Count1 : after(0.01,sec)
    Count1 -> Count2 : after(0.01,sec)
    Count2 -> Count3 : after(0.01,sec)
    Count3 -> Count4 : after(0.01,sec)
  data: RollingAliveCnt output double

== stateflow chart P2_SIL_Model_Diag/Controller/HSC/Camaro Fault Detection/Signal Generator /MCU_Signals/MCU_CAN_rolling/Rolling Alive Counter1 ==
  state RollingAliveCounter
    state Count1
      en: RollingAliveCnt=0
    state Count2
      en: RollingAliveCnt=1
    state Count3
      en: RollingAliveCnt=2
    state Count4
      en: RollingAliveCnt=3
    (default) -> Count1
    Count4 -> Count1 : after(0.01,sec)
    Count1 -> Count2 : after(0.01,sec)
    Count2 -> Count3 : after(0.01,sec)
    Count3 -> Count4 : after(0.01,sec)
  data: RollingAliveCnt output double

== stateflow chart P2_SIL_Model_Diag/Controller/HSC/Camaro Fault Detection/Signal Generator /TCM_Signals/TCM_Rolling/Rolling Alive Counter1 ==
  state RollingAliveCounter
    state Count1
      en: RollingAliveCnt=0
    state Count2
      en: RollingAliveCnt=1
    state Count3
      en: RollingAliveCnt=2
    state Count4
      en: RollingAliveCnt=3
    (default) -> Count1
    Count4 -> Count1 : after(0.01,sec)
    Count1 -> Count2 : after(0.01,sec)
    Count2 -> Count3 : after(0.01,sec)
    Count3 -> Count4 : after(0.01,sec)
  data: RollingAliveCnt output double

== stateflow chart P2_SIL_Model_Diag/Controller/HSC/Camaro Fault Detection/SystemDiag/Combined_SystemDiagnostics/Combined_System_Diagnostics ==
  state CombinedSystem_Online
    en: Combined_SystemStatus=2
  state Combined_System_Offline
    en:Combined_SystemStatus=0
  state Combined_System_Limited
    en: Combined_SystemStatus=1
  (default) -> Combined_System_Offline
  Combined_System_Offline -> CombinedSystem_Online [order 1] : [ECM_Status==2&&Clutch_Status==1&&Driver_Input_Status==1&&TCM_Status==2&&BMS_Status==2&&MCU_Status==2]
  CombinedSystem_Online -> Combined_System_Offline [order 1] : [Clutch_Status==0||ECM_Status==0||Driver_Input_Status==0||TCM_Status==0||BMS_Status==0||MCU_Status==0]
  Combined_System_Limited -> CombinedSystem_Online [order 2] : [ECM_Status==2&&Clutch_Status==1&&Driver_Input_Status==1&&TCM_Status==2&&BMS_Status==2&&MCU_Status==2]
  CombinedSystem_Online -> Combined_System_Limited [order 2] : [Driver_Input_Status==1&&Clutch_Status==1&&[ECM_Status==1||TCM_Status==1||BMS_Status==1||MCU_Status==1]]
  Combined_System_Limited -> Combined_System_Offline [order 1] : [Clutch_Status==0||ECM_Status==0||Driver_Input_Status==0||TCM_Status==0||BMS_Status==0||MCU_Status==0]
  Combined_System_Offline -> Combined_System_Limited [order 2] : [Driver_Input_Status==1&&Clutch_Status==1&&[ECM_Status==1||TCM_Status==1||BMS_Status==1||MCU_Status==1]]
  data: Driver_Input_Status input; BMS_Status input; MCU_Status input; ECM_Status input; TCM_Status input; Clutch_Status input; Combined_SystemStatus output

== stateflow chart P2_SIL_Model_Diag/Controller/HSC/Camaro Fault Detection/SystemDiag/eSystemDiagnostics/eSystem_Diagnostics ==
  state eSystem_Online
    en: eSystemStatus=2;
  state eSystem_Offline
    en:eSystemStatus=0;
  state eSystem_Limited
    en: eSystemStatus=1;
  (default) -> eSystem_Offline
  eSystem_Offline -> eSystem_Online [order 1] : [BMS_Status==2&&MCU_Status==2&&Driver_Input_Status==1&&TCM_Status==2]
  eSystem_Online -> eSystem_Offline [order 1] : [BMS_Status==0||MCU_Status==0||Driver_Input_Status==0||TCM_Status==0]
  eSystem_Online -> eSystem_Limited [order 2] : [Driver_Input_Status==1&&[BMS_Status==1||MCU_Status==1||TCM_Status==1]]
  eSystem_Limited -> eSystem_Online [order 2] : [BMS_Status==2&&MCU_Status==2&&Driver_Input_Status==1&&TCM_Status==2]
  eSystem_Limited -> eSystem_Offline [order 1] : [BMS_Status==0||MCU_Status==0||Driver_Input_Status==0||TCM_Status==0]
  eSystem_Offline -> eSystem_Limited [order 2] : [Driver_Input_Status==1&&[BMS_Status==1||MCU_Status==1||TCM_Status==1]]
  data: BMS_Status input; MCU_Status input; Driver_Input_Status input; TCM_Status input; eSystemStatus output

== stateflow chart P2_SIL_Model_Diag/Controller/HSC/Camaro Fault Detection/SystemDiag/iceSystemDiagnostics/iceSystem_Diagnostics ==
  state iceSystem_Online
    en: iceSystemStatus=2;
  state iceSystem_Offline
    en:iceSystemStatus=0;
  state iceSystem_Limited
    en: iceSystemStatus=1;
  (default) -> iceSystem_Offline
  iceSystem_Offline -> iceSystem_Online [order 1] : [ECM_Status==2&&Clutch_Status==1&&Driver_Input_Status==1&&TCM_Status==2]
  iceSystem_Online -> iceSystem_Offline [order 1] : [ECM_Status==0||Clutch_Status==0||Driver_Input_Status==0||TCM_Status==0]
  iceSystem_Online -> iceSystem_Limited [order 2] : [Driver_Input_Status==1&&Clutch_Status==1&&[ECM_Status==1||TCM_Status==1]]
  iceSystem_Limited -> iceSystem_Online [order 2] : [ECM_Status==2&&Clutch_Status==1&&Driver_Input_Status==1&&TCM_Status==2]
  iceSystem_Limited -> iceSystem_Offline [order 1] : [ECM_Status==0||Clutch_Status==0||Driver_Input_Status==0||TCM_Status==0]
  iceSystem_Offline -> iceSystem_Limited [order 2] : [Driver_Input_Status==1&&Clutch_Status==1&&(ECM_Status==1||TCM_Status==1)]
  data: ECM_Status input; Clutch_Status input; TCM_Status input; Driver_Input_Status input; iceSystemStatus output

== stateflow chart P2_SIL_Model_Diag/Controller/HSC/Camaro Fault Detection/Input Conversions/BMS_Conversions/BMS_rollingAliveCnt/Rolling Alive Counter ==
  state RollingAliveCounter
    state Count1
      en: RollingAliveCnt=0
    state Count2
      en: RollingAliveCnt=1
    state Count3
      en: RollingAliveCnt=2
    state Count4
      en: RollingAliveCnt=3
    (default) -> Count1
    Count4 -> Count1 : after(0.01,sec)
    Count1 -> Count2 : after(0.01,sec)
    Count2 -> Count3 : after(0.01,sec)
    Count3 -> Count4 : after(0.01,sec)
  data: RollingAliveCnt output double

== stateflow chart P2_SIL_Model_Diag/Controller/HSC/Camaro Fault Detection/Input Conversions/TCM_Conversions/TCM_Rolling/Rolling Alive Counter1 ==
  state RollingAliveCounter
    state Count1
      en: RollingAliveCnt=0;
    state Count2
      en: RollingAliveCnt=1;
    state Count3
      en: RollingAliveCnt=2;
    state Count4
      en: RollingAliveCnt=3;
    (default) -> Count1
    Count4 -> Count1 : after(0.01,sec)
    Count1 -> Count2 : after(0.01,sec)
    Count2 -> Count3 : after(0.01,sec)
    Count3 -> Count4 : after(0.01,sec)
  data: RollingAliveCnt output double

== stateflow chart P2_SIL_Model_Diag/Controller/HSC/Camaro Fault Detection/Input Conversions/Clutch_Conversions/Clutch_Rolling/Rolling Alive Counter1 ==
  state RollingAliveCounter
    state Count1
      en: RollingAliveCnt=0;
    state Count2
      en: RollingAliveCnt=1;
    state Count3
      en: RollingAliveCnt=2;
    state Count4
      en: RollingAliveCnt=3;
    (default) -> Count1
    Count4 -> Count1 : after(0.01,sec)
    Count1 -> Count2 : after(0.01,sec)
    Count2 -> Count3 : after(0.01,sec)
    Count3 -> Count4 : after(0.01,sec)
  data: RollingAliveCnt output double

== stateflow chart P2_SIL_Model_Diag/Camaro Plant Model/IMG/Soft MCU/MCU_CAN_rolling/Rolling Alive Counter1 ==
  state RollingAliveCounter
    state Count1
      en: RollingAliveCnt=0;
    state Count2
      en: RollingAliveCnt=1;
    state Count3
      en: RollingAliveCnt=2;
    state Count4
      en: RollingAliveCnt=3;
    (default) -> Count1
    Count4 -> Count1 : after(0.01,sec)
    Count1 -> Count2 : after(0.01,sec)
    Count2 -> Count3 : after(0.01,sec)
    Count3 -> Count4 : after(0.01,sec)
  data: RollingAliveCnt output double

== stateflow chart P2_SIL_Model_Diag/Camaro Plant Model/ESS/Soft BMS/RollingAliveCnt/Rolling Alive Counter ==
  state RollingAliveCounter
    state Count1
      en: RollingAliveCnt = 0;
    state Count2
      en: RollingAliveCnt = 1;
    state Count3
      en: RollingAliveCnt = 2;
    state Count4
      en: RollingAliveCnt = 3;
    (default) -> Count1
    Count4 -> Count1 : after(0.01,sec)
    Count1 -> Count2 : after(0.01,sec)
    Count2 -> Count3 : after(0.01,sec)
    Count3 -> Count4 : after(0.01,sec)
  data: RollingAliveCnt output int8 =0

== stateflow chart P2_SIL_Model_Diag/Controller/HSC/Camaro Fault Detection/Signal Diagnostic/Engine Signal Diagnostic/Rolling Alive Counter Detection1/Chart ==
  state Off
    en:flag=0;
  state Alive
    en:flag=1;
  state Dead
    en:flag=0;
  Alive -> Alive [order 1] : after(CycleTime-tloop,sec)
      | [PulseDetect==1]
  (default) -> Off
  Off -> Alive : [PulseDetect==1]
  Alive -> Dead [order 2] : after(CycleTime,sec)
  data: PulseDetect input; CycleTime input; flag output; tloop parameter

== stateflow chart P2_SIL_Model_Diag/Controller/HSC/Camaro Fault Detection/Signal Diagnostic/Transmission Signal Diagnostic/Rolling Alive Counter Detection/Chart ==
  state Off
    en:flag=0;
  state Alive
    en:flag=1;
  state Dead
    en:flag=0;
  Alive -> Alive [order 1] : after(CycleTime-tloop,sec)
      | [PulseDetect==1]
  (default) -> Off
  Off -> Alive : [PulseDetect==1]
  Alive -> Dead [order 2] : after(CycleTime,sec)
  data: PulseDetect input; CycleTime input; flag output; tloop parameter
